simulink model "untitled"  (R2023a)
settings: Solver=VariableStepDiscrete  StartTime=0.0  StopTime=Ta  MaxStep=0.1  RelTol=1e-3
libraries: simulink x3, dsparch4 x1
settings Model: Creator=alexis  LastModifiedBy=alexis

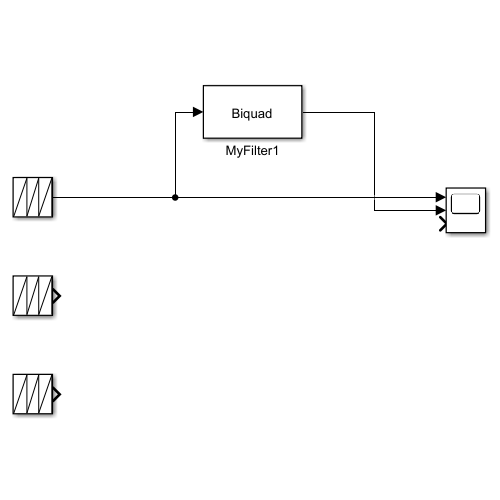
[thumbnail: Simulink's stored preview of the top-level diagram]
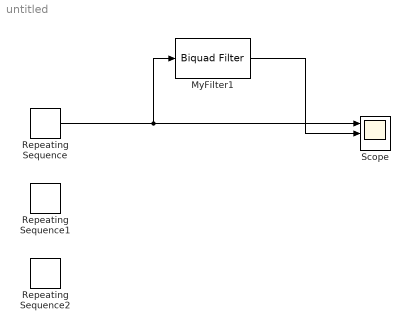
== system untitled ==
  MyFilter1 : dsparch4/Biquad Filter  Tag=BlockMethodSubSystem  FilterSource=Dialog parameters  CoeffSource=Specify via dialog  FilterObject=BQF  IIRFiltStruct=Direct form II  BiQuadCoeffs=[1 -1.49838269063269558 1 1 -1.61532430425266216 0.962192137724845797;1 -1.37427325100254838 1 1 -1.64208328743736987 0.914340755835776231;1 -0.949983471868511953 1 1 -1.68985988950789756 0.840190372476980252;1 0.872353434164175989 1 1 -1.73573894930548844 0.771009251186532851;1 -1.53699031762575045 1 1 -1.61002347483199215 0.989596397046260345]  ScaleValues=[0.734170117209946183;0.712706105090281872;0.493995620630140186;0.372067034048319811;0.00401848626225551585;1]  IC=0  ICnum=0  ICden=0  a0Flag=Warning  optimizeScaleValues=on  ScaleValueMode=Specify via input port (g)  roundingMode=Floor  overflowMode=off  scaleValueFracLength=14  denProdOutputFracLength=30  denAccumFracLength=30  secondMemoryFracLength=15
  Repeating Sequence : simulink/Sources/Repeating Sequence  rep_seq_t=T  rep_seq_y=X
  Repeating Sequence1 : simulink/Sources/Repeating Sequence  rep_seq_t=T  rep_seq_y=Y
  Repeating Sequence2 : simulink/Sources/Repeating Sequence  rep_seq_t=T  rep_seq_y=Z
  Scope : Scope  NumInputPorts=3
  wires:
  Repeating Sequence/1 -> MyFilter1/1, Scope/1
  MyFilter1/1 -> Scope/2
